simulink model "sensordata_group"  (Simulink 9.1)
settings: Solver=VariableStepAuto  StartTime=0.0  StopTime=10.0  RelTol=1e-3
libraries: F_Line_block x11
settings Model: LogicAnalyzerSignalOrdering=6fbe5520-670a-4c18-be9e-55fb81ad124d  Creator=dongw  LastModifiedBy=dongw
settings DataIOCC: SaveFormat=Dataset
settings OptimizationCC: LifeSpan=auto
settings DebuggingCC: UnderspecifiedInitializationDetection=Simplified  MergeDetectMultiDrivingBlocksExec=error  SFUnexpectedBacktrackingDiag=error  SFNoUnconditionalDefaultTransitionDiag=error  SFExecutionAtInitializationDiag=warning
settings HardwareCC: ProdBitPerPointer=64  ProdBitPerSizeT=64  ProdBitPerPtrDiffT=64  ProdLargestAtomicFloat=Float  ProdIntDivRoundTo=Zero  ProdEndianess=LittleEndian  ProdWordSize=64  ProdHWDeviceType=Intel->x86-64 (Windows64)
settings ModelReferenceCC: PropagateSignalLabelsOutOfModel=on
settings CodeAppCC: StateflowObjectComments=off
settings GRTTargetCC: TargetLangStandard=C99 (ISO)  CombineOutputUpdateFcns=on  GRTInterface=off
settings ConfigComp: CovMetricSettings=dwe  CovHtmlReporting=off  CovSaveCumulativeToWorkspaceVar=off  CovSaveSingleToWorkspaceVar=off  CovExternalEMLEnable=on

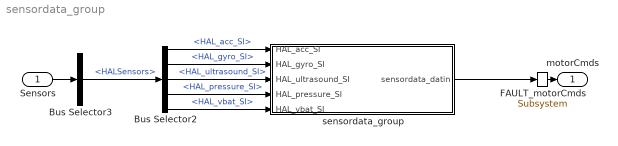
== system sensordata_group ==
  Sensors : Inport  OutDataTypeStr=Bus: SensorsBus  BusOutputAsStruct=on
  Bus Selector2 : BusSelector  OutputSignals=HAL_acc_SI,HAL_gyro_SI,HAL_ultrasound_SI,HAL_pressure_SI,HAL_vbat_SI
  Bus Selector3 : BusSelector  OutputSignals=HALSensors
  sensordata_group : Subsystem
  motorCmds : Outport
  FAULT_motorCmds : F_Line_block/Subsystem
  wires:
  Bus Selector2/4 -> sensordata_group/4(HAL_pressure_SI)  "<HAL_pressure_SI>"
  Bus Selector2/5 -> sensordata_group/5(HAL_vbat_SI)  "<HAL_vbat_SI>"
  Bus Selector2/1 -> sensordata_group/1(HAL_acc_SI)  "<HAL_acc_SI>"
  Bus Selector2/2 -> sensordata_group/2(HAL_gyro_SI)  "<HAL_gyro_SI>"
  Sensors/1 -> Bus Selector3/1
  Bus Selector3/1 -> Bus Selector2/1  "<HALSensors>"
  Bus Selector2/3 -> sensordata_group/3(HAL_ultrasound_SI)  "<HAL_ultrasound_SI>"
  sensordata_group/1(sensordata_datin) -> FAULT_motorCmds/1
  FAULT_motorCmds/1 -> motorCmds/1

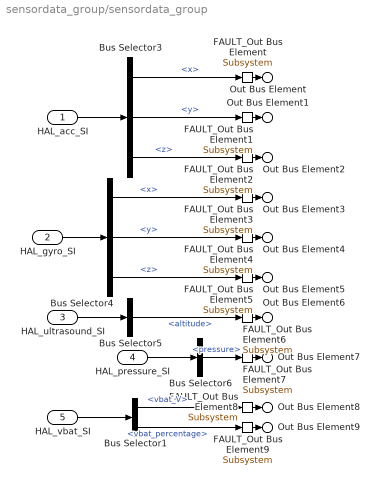
== system sensordata_group/sensordata_group ==
  HAL_acc_SI : Inport  OutDataTypeStr=Bus: HAL_acc_SI_t
  HAL_gyro_SI : Inport  Port=2  OutDataTypeStr=Bus: HAL_gyro_SI_t
  HAL_ultrasound_SI : Inport  Port=3  OutDataTypeStr=Bus: HAL_ultrasound_SI_t
  HAL_pressure_SI : Inport  Port=4  OutDataTypeStr=Bus: HAL_pressure_SI_t
  HAL_vbat_SI : Inport  Port=5  OutDataTypeStr=Bus: HAL_vbat_SI_t
  Bus Selector1 : BusSelector  OutputSignals=vbat_V,vbat_percentage
  Bus Selector3 : BusSelector  OutputSignals=x,y,z
  Bus Selector4 : BusSelector  OutputSignals=x,y,z
  Bus Selector5 : BusSelector  OutputSignals=altitude
  Bus Selector6 : BusSelector  OutputSignals=pressure
  Out Bus Element : Outport  PortName=sensordata_datin  Element=ddx
  FAULT_Out Bus Element{,1..9} (10 alike) : F_Line_block/Subsystem
  Out Bus Element1 : Outport  PortName=sensordata_datin  Element=ddy
  Out Bus Element2 : Outport  PortName=sensordata_datin  Element=ddz
  Out Bus Element3 : Outport  PortName=sensordata_datin  Element=p
  Out Bus Element4 : Outport  PortName=sensordata_datin  Element=q
  Out Bus Element5 : Outport  PortName=sensordata_datin  Element=r
  Out Bus Element6 : Outport  PortName=sensordata_datin  Element=altitude_sonar
  Out Bus Element7 : Outport  PortName=sensordata_datin  Element=prs
  Out Bus Element8 : Outport  PortName=sensordata_datin  Element=vbat_V
  Out Bus Element9 : Outport  PortName=sensordata_datin  Element=vbat_percentage
  wires:
  HAL_gyro_SI/1 -> Bus Selector4/1
  HAL_acc_SI/1 -> Bus Selector3/1
  HAL_pressure_SI/1 -> Bus Selector6/1
  HAL_ultrasound_SI/1 -> Bus Selector5/1
  Bus Selector4/1 -> FAULT_Out Bus Element3/1  "<x>"
  FAULT_Out Bus Element3/1 -> Out Bus Element3/1
  Bus Selector3/3 -> FAULT_Out Bus Element2/1  "<z>"
  FAULT_Out Bus Element2/1 -> Out Bus Element2/1
  Bus Selector4/3 -> FAULT_Out Bus Element5/1  "<z>"
  FAULT_Out Bus Element5/1 -> Out Bus Element5/1
  Bus Selector5/1 -> FAULT_Out Bus Element6/1  "<altitude>"
  FAULT_Out Bus Element6/1 -> Out Bus Element6/1
  Bus Selector6/1 -> FAULT_Out Bus Element7/1  "<pressure>"
  FAULT_Out Bus Element7/1 -> Out Bus Element7/1
  Bus Selector4/2 -> FAULT_Out Bus Element4/1  "<y>"
  FAULT_Out Bus Element4/1 -> Out Bus Element4/1
  Bus Selector3/1 -> FAULT_Out Bus Element/1  "<x>"
  FAULT_Out Bus Element/1 -> Out Bus Element/1
  Bus Selector3/2 -> FAULT_Out Bus Element1/1  "<y>"
  FAULT_Out Bus Element1/1 -> Out Bus Element1/1
  Bus Selector1/1 -> FAULT_Out Bus Element8/1  "<vbat_V>"
  FAULT_Out Bus Element8/1 -> Out Bus Element8/1
  HAL_vbat_SI/1 -> Bus Selector1/1
  Bus Selector1/2 -> FAULT_Out Bus Element9/1  "<vbat_percentage>"
  FAULT_Out Bus Element9/1 -> Out Bus Element9/1
